simulink model "ControleSMRG"  (R2020a)
settings: Solver=FixedStepAuto  StartTime=0.0  StopTime=10000  FixedStep=0.1  RelTol=1e-3
settings Model: Creator=altop  LastModifiedBy=victo

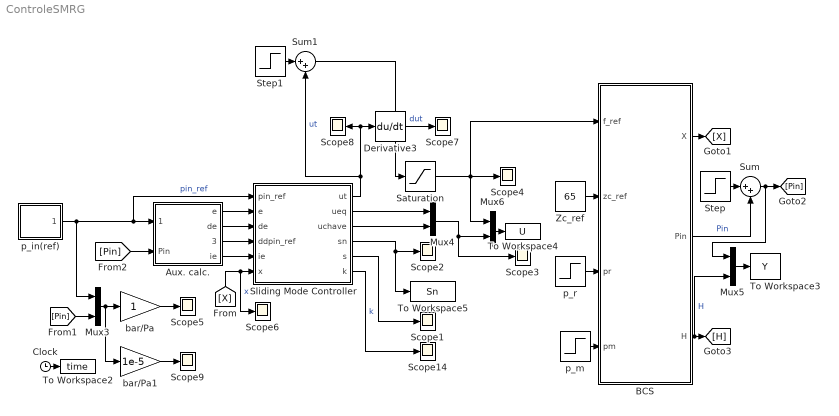
== system ControleSMRG ==
  Aux. calc. : Subsystem
  BCS : Subsystem
      mask Display: image('$imagefile'); % Use "Edit Image" on toolstrip to change.
  Clock : Clock
      settings: Decimation=15
  Derivative3 : Derivative
  Mux{3..6} (4 alike) : Mux  Inputs=2
  Saturation : Saturate  UpperLimit=65  LowerLimit=35
  Scope{1..9,14} (10 alike) : Scope
  Sliding Mode Controller : Subsystem  mask{lambda=6, delta=5e5, eta=0, PI_n=2.0e-09, rho_n=809, mu_n=0.045, IN=incerteza total (PI,\mu,\rho)}
      mask prompts: lambda "\lambda"; delta "\delta"; eta "\eta"; PI_n "PI"; rho_n "\rho"; mu_n "\mu"; IN "Caso"
      mask TypeOptions IN: incerteza em PI | incerteza em \mu | incerteza em \rho | incerteza total (PI,\mu,\rho) | Nominal
      mask DialogControl DescGroupVar Prompt: Integral Action Slinding Mode Control
      mask DialogControl Container3 Prompt: Control Tunning
  Step : Step  Time=11000  After=1e5  SampleTime=0
  Step1 : Step  Time=11000  After=8  SampleTime=0
  Sum : Sum  Inputs=|++
  Sum1 : Sum  Inputs=|++
  To Workspace2 : ToWorkspace  VariableName=time  SampleTime=-1
      settings: Save2DSignal=2-D array (concatenate along first dimension)
  To Workspace3 : ToWorkspace  VariableName=Y  SampleTime=-1
  To Workspace4 : ToWorkspace  VariableName=U  SampleTime=-1
  To Workspace5 : ToWorkspace  VariableName=Sn  SampleTime=-1
  Zc_ref : Constant  Value=65
  bar/Pa : Gain
  bar/Pa1 : Gain  Gain=1e-5
  p_in(ref) : Subsystem
  p_m : Step  Time=11000  Before=2e5  After=2e6  SampleTime=0
  p_r : Step  Time=11000  Before=1.26e7  After=1.20e7  SampleTime=0
  wires:
  Clock/1 -> To Workspace2/1
  Saturation/1 -> Mux6/1, BCS/1(f_ref), Scope4/1
  Mux3/1 -> bar/Pa1/1, bar/Pa/1
  Mux4/1 -> Mux6/2, Scope3/1
  bar/Pa/1 -> Scope5/1
  Derivative3/1 -> Scope7/1  "dut"
  Mux6/1 -> To Workspace4/1
  p_in(ref)/1(pin_ref) -> Aux. calc./1(pin_ref), Sliding Mode Controller/1(pin_ref), Mux3/1  "pin_ref"
  [Pin] -> Mux3/2
  Sliding Mode Controller/4(sn) -> To Workspace5/1, Scope2/1
  Sliding Mode Controller/1(ut) -> Sum1/2, Scope8/1, Derivative3/1  "ut"
  [X] -> Scope6/1, Sliding Mode Controller/6(x)  "x"
  Sliding Mode Controller/2(ueq) -> Mux4/1
  Sliding Mode Controller/3(uchave) -> Mux4/2
  Sliding Mode Controller/5(s) -> Scope1/1
  Sliding Mode Controller/6(k) -> Scope14/1  "k"
  BCS/1(X) -> [X]
  [Pin] -> Aux. calc./2(Pin)
  Aux. calc./1(e) -> Sliding Mode Controller/2(e)
  Aux. calc./2(de) -> Sliding Mode Controller/3(de)
  Aux. calc./4(ie) -> Sliding Mode Controller/5(ie)
  Aux. calc./3(ddpin_ref) -> Sliding Mode Controller/4(ddpin_ref)
  Zc_ref/1 -> BCS/2(zc_ref)
  p_r/1 -> BCS/3(pr)
  p_m/1 -> BCS/4(pm)
  bar/Pa1/1 -> Scope9/1
  Step/1 -> Sum/1
  Step1/1 -> Sum1/1
  Sum1/1 -> Saturation/1
  BCS/3(H) -> Mux5/2, [H]  "H"
  Mux5/1 -> To Workspace3/1
  BCS/2(Pin) -> Sum/2  "Pin"
  Sum/1 -> Mux5/1, [Pin]

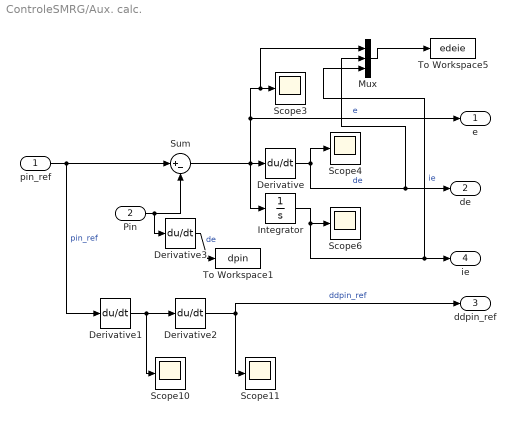
== system ControleSMRG/Aux. calc. ==
  pin_ref : Inport
  Pin : Inport  Port=2
  Derivative{,1..3} (4 alike) : Derivative
  Integrator : Integrator
  Mux : Mux  Inputs=3
  Scope{3..4,6,10..11} (5 alike) : Scope
  Sum : Sum  Inputs=|+-
  To Workspace1 : ToWorkspace  VariableName=dpin  SampleTime=-1
  To Workspace5 : ToWorkspace  VariableName=edeie  SampleTime=-1
  e : Outport
  de : Outport  Port=2
  ddpin_ref : Outport  Port=3
  ie : Outport  Port=4
  wires:
  Sum/1 -> e/1, Mux/1, Scope3/1, Integrator/1, Derivative/1  "e"
  Derivative/1 -> Mux/2, de/1, Scope4/1  "de"
  Pin/1 -> Derivative3/1, Sum/2
  Integrator/1 -> Mux/3, ie/1, Scope6/1  "ie"
  pin_ref/1 -> Sum/1, Derivative1/1  "pin_ref"
  Derivative2/1 -> Scope11/1, ddpin_ref/1  "ddpin_ref"
  Derivative1/1 -> Derivative2/1, Scope10/1
  Mux/1 -> To Workspace5/1
  Derivative3/1 -> To Workspace1/1  "de"

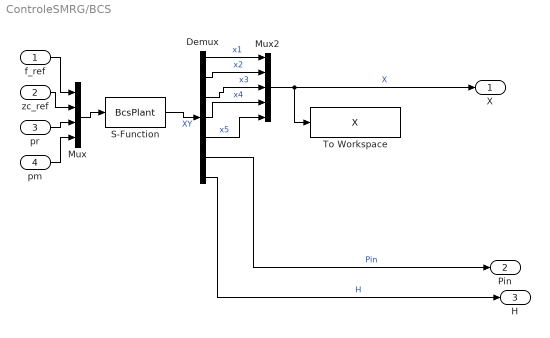
== system ControleSMRG/BCS ==
  f_ref : Inport
  zc_ref : Inport  Port=2
  pr : Inport  Port=3
  pm : Inport  Port=4
  Demux : Demux  Outputs=7
  Mux : Mux
  Mux2 : Mux  Inputs=5
  S-Function : S-Function  FunctionName=BcsPlant  SFunctionDeploymentMode=off  EnableBusSupport=off
  To Workspace : ToWorkspace  VariableName=X  SampleTime=-1
  X : Outport
  Pin : Outport  Port=2
  H : Outport  Port=3
  wires:
  Demux/3 -> Mux2/3  "x3"
  Demux/5 -> Mux2/5  "x5"
  Demux/4 -> Mux2/4  "x4"
  Demux/1 -> Mux2/1  "x1"
  Demux/2 -> Mux2/2  "x2"
  Mux2/1 -> X/1, To Workspace/1  "X"
  f_ref/1 -> Mux/1
  Demux/7 -> H/1  "H"
  Demux/6 -> Pin/1  "Pin"
  S-Function/1 -> Demux/1  "XY"
  Mux/1 -> S-Function/1
  zc_ref/1 -> Mux/2
  pr/1 -> Mux/3
  pm/1 -> Mux/4

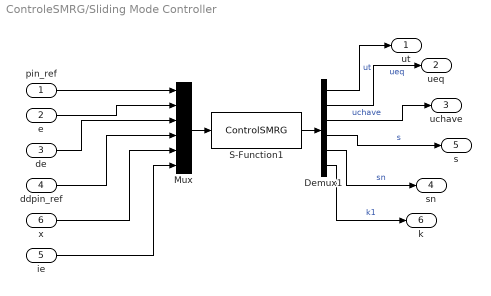
== system ControleSMRG/Sliding Mode Controller ==
  pin_ref : Inport
  e : Inport  Port=2
  de : Inport  Port=3
  ddpin_ref : Inport  Port=4
  ie : Inport  Port=5
  x : Inport  Port=6
  Demux1 : Demux  Outputs=6
  Mux : Mux  Inputs=6
  S-Function1 : S-Function  FunctionName=ControlSMRG  Parameters=PI_n,rho_n,mu_n,lambda,delta,eta,IN  SFunctionDeploymentMode=off  EnableBusSupport=off
  ut : Outport
  ueq : Outport  Port=2
  uchave : Outport  Port=3
  sn : Outport  Port=4
  s : Outport  Port=5
  k : Outport  Port=6
  wires:
  Mux/1 -> S-Function1/1
  ddpin_ref/1 -> Mux/4
  Demux1/6 -> k/1  "k1"
  Demux1/2 -> ueq/1  "ueq"
  Demux1/4 -> s/1  "s"
  S-Function1/1 -> Demux1/1
  de/1 -> Mux/3
  pin_ref/1 -> Mux/1
  ie/1 -> Mux/6
  Demux1/1 -> ut/1  "ut"
  Demux1/5 -> sn/1  "sn"
  Demux1/3 -> uchave/1  "uchave"
  e/1 -> Mux/2
  x/1 -> Mux/5

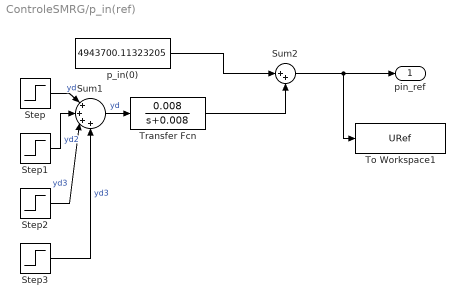
== system ControleSMRG/p_in(ref) ==
  Step : Step  Time=500  After=-17e5  SampleTime=0
  Step1 : Step  Time=2500  After=8e5  SampleTime=0
  Step2 : Step  Time=5000  After=13e5  SampleTime=0
  Step3 : Step  Time=8000  After=9e5  SampleTime=0
  Sum1 : Sum  Inputs=|++++
  Sum2 : Sum  Inputs=|++
  To Workspace1 : ToWorkspace  VariableName=URef  SampleTime=-1
  Transfer Fcn : TransferFcn  Numerator=[0.008]  Denominator=[1 0.008]
  p_in(0) : Constant  Value=4943700.11323205
  pin_ref : Outport
  wires:
  Step1/1 -> Sum1/2  "yd2"
  p_in(0)/1 -> Sum2/1
  Sum1/1 -> Transfer Fcn/1  "yd"
  Step2/1 -> Sum1/3  "yd3"
  Step3/1 -> Sum1/4  "yd3"
  Step/1 -> Sum1/1  "yd"
  Transfer Fcn/1 -> Sum2/2
  Sum2/1 -> To Workspace1/1, pin_ref/1
